simulink model "hostComms"  (R2014b)
settings: Solver=ode45  StartTime=0.0  StopTime=10.0  RelTol=1e-3
undefined symbols (not defined in the file or in its folder): gcbh, rmidispblock
libraries: hostLib x1
settings Model: DataDictionary=hostData.sldd  Creator=scastro  LastModifiedBy=scastro

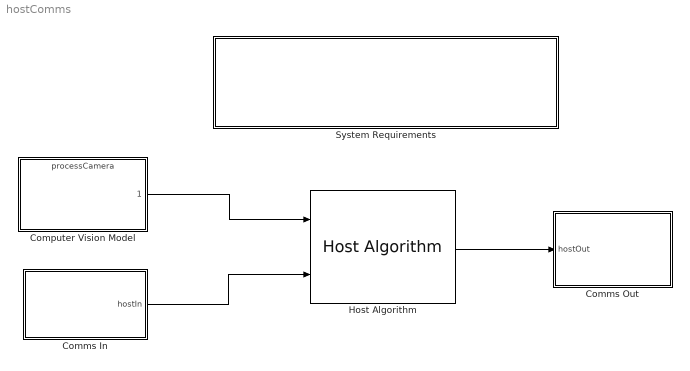
== system hostComms ==
  Comms In : Subsystem
  Comms Out : Subsystem
  Computer Vision Model : ModelReference  ModelNameDialog=processCamera  SimulationMode=Normal  ModelReferenceVersion=1.2  CopyOfModelName=processCamera  DefaultDataLogging=on
  Host Algorithm : hostLib/Host Algorithm
  System Requirements : Subsystem  LoadFcn=rmidispblock('load',gcbh)  mask(System Requirements){id=SystemReq, title=System Requirements}
      mask prompts: title "Block Title"
      mask help: Lists the requirements for the current model.
      mask init:
      | id = 'SystemReq';
      | [w,h] = rmidispblock('display',gcbh);
      settings: CopyFcn=rmidispblock('create',gcbh)  DeleteFcn=rmidispblock('delete',gcbh)  ModelCloseFcn=rmidispblock('close',gcbh)  PreSaveFcn=rmidispblock('close',gcbh)  PostSaveFcn=rmidispblock('open',gcbh)  OpenFcn=rmidispblock('open',gcbh)  MoveFcn=rmidispblock('move',gcbh)
      mask Help: helpview(fullfile(docroot,'toolbox','slvnv','slvnv.map'),'systemrequirements')
      mask Display:
      | text(341/2,88-4,rmidispblock('title',gcbh),'horizontalAlignment','center','verticalAlignment','top')
      | text(w/2,h/2,'<No Requirements in System>','horizontalAlignment','center','verticalAlignment','top')
  wires:
  Computer Vision Model/1 -> Host Algorithm/1
  Comms In/1(hostIn) -> Host Algorithm/2
  Host Algorithm/1 -> Comms Out/1(hostOut)

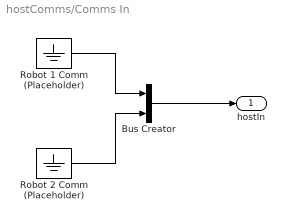
== system hostComms/Comms In ==
  Bus Creator : BusCreator  Inputs=2
  Robot 1 Comm (Placeholder) : Ground
  Robot 2 Comm (Placeholder) : Ground
  hostIn : Outport
  wires:
  Bus Creator/1 -> hostIn/1
  Robot 1 Comm (Placeholder)/1 -> Bus Creator/1
  Robot 2 Comm (Placeholder)/1 -> Bus Creator/2

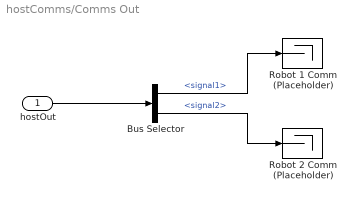
== system hostComms/Comms Out ==
  hostOut : Inport
  Bus Selector : BusSelector  OutputSignals=signal1,signal2
  Robot 1 Comm (Placeholder) : Terminator
  Robot 2 Comm (Placeholder) : Terminator
  wires:
  Bus Selector/2 -> Robot 2 Comm (Placeholder)/1  "<signal2>"
  hostOut/1 -> Bus Selector/1
  Bus Selector/1 -> Robot 1 Comm (Placeholder)/1  "<signal1>"

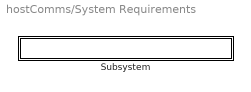
== system hostComms/System Requirements ==
  Subsystem : Subsystem  mask{label=0, index=1}
      mask init:
      | label = rmidispblock('label',index);
      settings: OpenFcn=rmidispblock('openReq',gcbh);
      mask Display: text(0,0,label,'horizontalAlignment','left','verticalAlignment','bottom')

== system hostComms/System Requirements/Subsystem ==
